simulink model "SIRV_V2"  (R2023b)
settings: Solver=VariableStepAuto  StartTime=0.0  StopTime=10.0  RelTol=1e-3
undefined symbols (not defined in the file): B, Beta_, d, gamma_, nu_, p
settings Model: Creator=simon  LastModifiedBy=simon

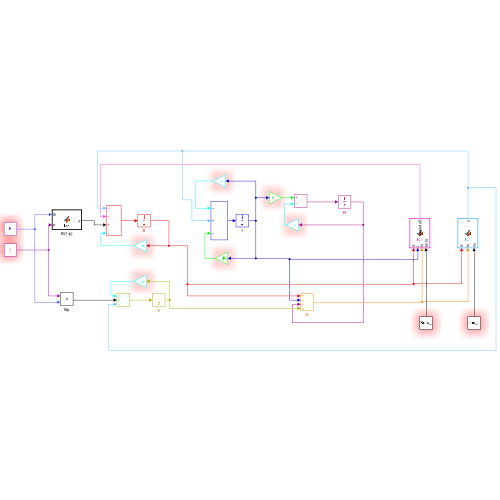
[thumbnail: Simulink's stored preview of the top-level diagram]
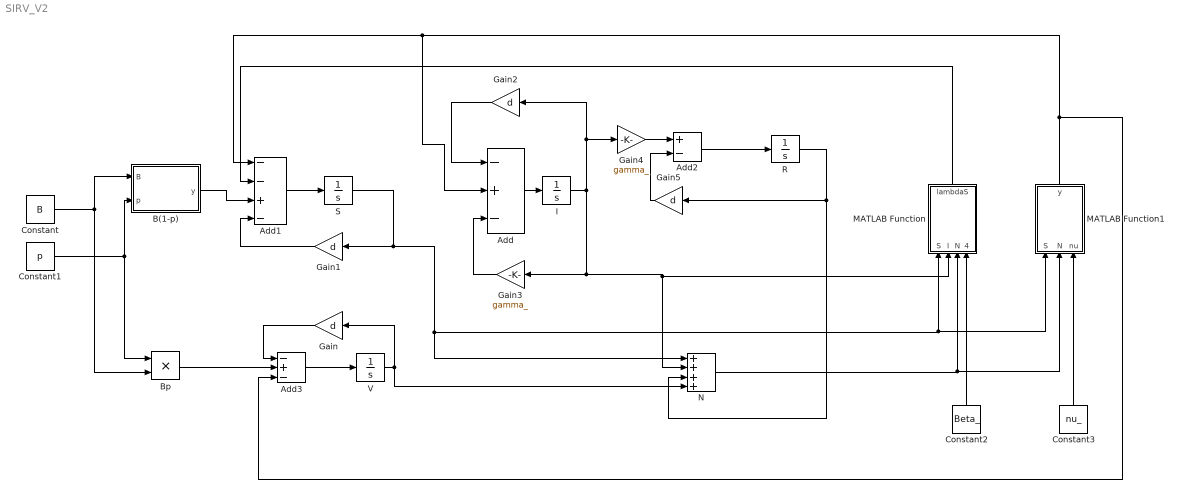
== system SIRV_V2 ==
  Add : Sum  Inputs=-+-
  Add1 : Sum  Inputs=--+-
  Add2 : Sum  Inputs=+-
  Add3 : Sum  Inputs=-+-
  B(1-p) : MATLAB Function  TreatAsAtomicUnit=on
  Bp : Product
  Constant : Constant  Value=B
  Constant1 : Constant  Value=p
  Constant2 : Constant  Value=Beta_
  Constant3 : Constant  Value=nu_
  Gain{,1..2,5} (4 alike) : Gain  Gain=d
  Gain3 : Gain  Gain=gamma_
  Gain4 : Gain  Gain=gamma_
  I : Integrator
  MATLAB Function : MATLAB Function  TreatAsAtomicUnit=on
  MATLAB Function1 : MATLAB Function  TreatAsAtomicUnit=on
  N : Sum  Inputs=++++
  R : Integrator
  S : Integrator
  V : Integrator
  wires:
  Add/1 -> I/1
  Add2/1 -> R/1
  Add3/1 -> V/1
  R/1 -> N/3, Gain5/1
  Add1/1 -> S/1
  V/1 -> N/4, Gain/1
  Constant/1 -> B(1-p)/1(B), Bp/2
  Constant1/1 -> Bp/1, B(1-p)/2(p)
  B(1-p)/1(y) -> Add1/3
  Bp/1 -> Add3/2
  Gain/1 -> Add3/1
  Gain1/1 -> Add1/4
  Gain2/1 -> Add/1
  Gain3/1 -> Add/3
  Gain4/1 -> Add2/1
  Gain5/1 -> Add2/2
  Constant2/1 -> MATLAB Function/4(beta)
  MATLAB Function/1(lambdaS) -> Add1/2
  I/1 -> Gain2/1, Gain4/1, MATLAB Function/2(I), N/2, Gain3/1
  Constant3/1 -> MATLAB Function1/3(nu)
  N/1 -> MATLAB Function1/2(N), MATLAB Function/3(N)
  S/1 -> MATLAB Function1/1(S), MATLAB Function/1(S), N/1, Gain1/1
  MATLAB Function1/1(y) -> Add3/3, Add/2, Add1/1

== matlab function SIRV_V2/MATLAB Function ==
  data: S input; I input; N input; beta input; lambdaS output
function lambdaS = fcn(S,I,N,beta)

lambdaS = S*((beta*I)/N);

== matlab function SIRV_V2/B(1-p) ==
  data: B input; y output; p input
function y = fcn(B,p)

y = B(1-p);

== matlab function SIRV_V2/MATLAB Function1 ==
  data: S input; N input; nu input; y output
function y = fcn(S,N,nu)

y = (nu*S)/N;
